simulink library "halout"  (R2021b)
settings: Solver=VariableStepAuto  StartTime=0.0  StopTime=10.0  RelTol=1e-3
undefined symbols (not defined in the file): C_TASK_5MS_S, FALSE, KHAL_CAN1FDAPS3E2E_flg, KHAL_CAN1FDAPS3TxReq_flg, KHAL_CAN1FDVCU2E2E_flg, KHAL_CAN1FDVCU2TxReq_flg, KHAL_CAN1FDVCU3E2E_flg, KHAL_CAN1FDVCU3TxReq_flg, KHAL_CAN1TxReq_flg, KHAL_CAN2TxReq_flg, KHAL_CAN3FDVCU1TxReq_flg, KHAL_CAN3FDVCU2E2E_flg, KHAL_CAN3FDVCU2TxReq_flg, KHAL_CAN3TxReq_flg, KHAL_CAN4FDVCU1E2E_flg, KHAL_CAN4FDVCU1TxReq_flg, KHAL_CAN4TxReq_flg, KHAL_CAN5TxReq_flg, ONE_INT, TRUE, ZERO_INT
libraries: FVT_lib x383, simulink x179
(part 1 of 20)
settings Model: Creator=13168  LastModifiedBy=yenst
settings SolverCC: AlgebraicLoopSolver=TrustRegion
settings DataIOCC: SaveFormat=Array  SignalLoggingSaveFormat=ModelDataLogs  ReturnWorkspaceOutputs=off
settings OptimizationCC: BlockReduction=off  BooleanDataType=off
settings DebuggingCC: SaveWithParameterizedLinksMsg=none  UnderspecifiedInitializationDetection=Classic  MergeDetectMultiDrivingBlocksExec=none  SignalResolutionControl=TryResolveAllWithWarning  SFMachineParentedDataDiag=warning
settings HardwareCC: TargetUnknown=on
settings ModelReferenceCC: PropagateSignalLabelsOutOfModel=off
settings ConfigComp: CovMetricSettings=dw  CovSaveCumulativeToWorkspaceVar=on  CovSaveSingleToWorkspaceVar=on

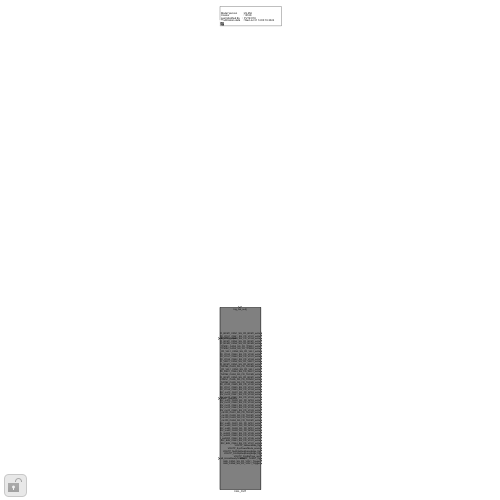
[thumbnail: Simulink's stored preview of the top-level diagram]
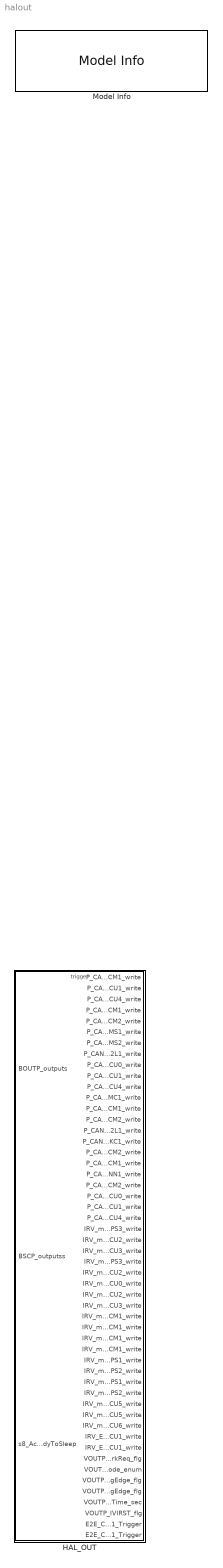
== system halout ==
  HAL_OUT : Subsystem
      settings: RTWSystemCode=Nonreusable function  RTWFcnNameOpts=Use subsystem name  RTWFileNameOpts=Use subsystem name
  Model Info : simulink/Model-Wide Utilities/Model Info  Frame=on  DisplayStringWithTags=|  HorizontalTextAlignment=Left  LeftAlignmentValue=0.02
      | Model Version        : %<ModelVersion>
      | Creator                   : %<Creator>
      | Last Modified By    : %<LastModifiedBy>
      | Modification date    : %<LastModificationDate>

== system halout/HAL_OUT ==
  BOUTP_outputs : Inport  OutDataTypeStr=Bus: BOUTP_outputs
  BSCP_outputss : Inport  Port=2  OutDataTypeStr=Bus:BSCP_outputs
  s8_AcoreReadyToSleep : Inport  Port=3
  trig_hal_out : TriggerPort  TriggerType=function-call  VariantControl=(inherit)
  Bus Selector : BusSelector  OutputSignals=VOUTP_AllCANTxReq_flg
  Bus_Selector : BusSelector  OutputSignals=VOUTP_NetworkReq_flg,VOUTP_SysPowerMode_enum,VOUTP_NvWriteReqRisingEdge_flg,VOUTP_FdcSlpReqRisingEdge_flg,VOUTP_FdcSlpTime_sec,VOUTP_IVIRST_flg
  CAN1 : Subsystem  TreatAsAtomicUnit=on
  CAN2 : Subsystem  TreatAsAtomicUnit=on
  CAN3 : Subsystem  TreatAsAtomicUnit=on
  CAN4 : Subsystem  TreatAsAtomicUnit=on
  CAN5 : Subsystem  TreatAsAtomicUnit=on
  CAN_Scheduler : Stateflow chart  TreatAsAtomicUnit=on
  Constant : Constant  Value=KHAL_CAN1TxReq_flg
  Constant1 : Constant  Value=KHAL_CAN2TxReq_flg
  Constant2 : Constant  Value=KHAL_CAN3TxReq_flg
  Constant3 : Constant  Value=KHAL_CAN4TxReq_flg
  Constant4 : Constant  Value=KHAL_CAN5TxReq_flg
  P_CAN1_FD_BCM1_CAN1_SG_FD_BCM1_write : Outport  OutDataTypeStr=Bus: DT_CAN1_SG_FD_BCM1
  P_CAN1_FD_VCU1_CAN1_SG_FD_VCU1_write : Outport  Port=2  OutDataTypeStr=Bus: DT_CAN1_SG_FD_VCU1
  P_CAN1_FD_VCU4_CAN1_SG_FD_VCU4_write : Outport  Port=3  OutDataTypeStr=Bus: DT_CAN1_SG_FD_VCU4
  P_CAN2_FD_BCM1_CAN2_SG_FD_BCM1_write : Outport  Port=4  OutDataTypeStr=Bus: DT_CAN2_SG_FD_BCM1
  P_CAN2_FD_BCM2_CAN2_SG_FD_BCM2_write : Outport  Port=5  OutDataTypeStr=Bus: DT_CAN2_SG_FD_BCM2
  P_CAN2_FD_TPMS1_CAN2_SG_FD_TPMS1_write : Outport  Port=6  OutDataTypeStr=Bus: DT_CAN2_SG_FD_TPMS1
  P_CAN2_FD_TPMS2_CAN2_SG_FD_TPMS2_write : Outport  Port=7  OutDataTypeStr=Bus: DT_CAN2_SG_FD_TPMS2
  P_CAN2_FD_V2L1_CAN2_SG_FD_V2L1_write : Outport  Port=8  OutDataTypeStr=Bus: DT_CAN2_SG_FD_V2L1
  P_CAN2_FD_VCU0_CAN2_SG_FD_VCU0_write : Outport  Port=9  OutDataTypeStr=Bus: DT_CAN2_SG_FD_VCU0
  P_CAN2_FD_VCU1_CAN2_SG_FD_VCU1_write : Outport  Port=10  OutDataTypeStr=Bus: DT_CAN2_SG_FD_VCU1
  P_CAN2_FD_VCU4_CAN2_SG_FD_VCU4_write : Outport  Port=11  OutDataTypeStr=Bus: DT_CAN2_SG_FD_VCU4
  P_CAN2_FD_VMC1_CAN2_SG_FD_VMC1_write : Outport  Port=12  OutDataTypeStr=Bus: DT_CAN2_SG_FD_VMC1
  P_CAN3_FD_BCM1_CAN3_SG_FD_BCM1_write : Outport  Port=13  OutDataTypeStr=Bus: DT_CAN3_SG_FD_BCM1
  P_CAN3_FD_THCM2_CAN3_SG_FD_THCM2_write : Outport  Port=14  OutDataTypeStr=Bus: DT_CAN3_SG_FD_THCM2
  P_CAN3_FD_V2L1_CAN3_SG_FD_V2L1_write : Outport  Port=15  OutDataTypeStr=Bus: DT_CAN3_SG_FD_V2L1
  P_CAN4_FD_DKC1_CAN4_SG_FD_DKC1_write : Outport  Port=16  OutDataTypeStr=Bus: DT_CAN4_SG_FD_DKC1
  P_CAN4_FD_THCM2_CAN4_SG_FD_THCM2_write : Outport  Port=17  OutDataTypeStr=Bus: DT_CAN4_SG_FD_THCM2
  P_CAN5_FD_BCM1_CAN5_SG_FD_BCM1_write : Outport  Port=18  OutDataTypeStr=Bus: DT_CAN5_SG_FD_BCM1
  P_CAN5_FD_CONN1_CAN5_SG_FD_CONN1_write : Outport  Port=19  OutDataTypeStr=Bus: DT_CAN5_SG_FD_CONN1
  P_CAN5_FD_THCM2_CAN5_SG_FD_THCM2_write : Outport  Port=20  OutDataTypeStr=Bus: DT_CAN5_SG_FD_THCM2
  P_CAN5_FD_VCU0_CAN5_SG_FD_VCU0_write : Outport  Port=21  OutDataTypeStr=Bus: DT_CAN5_SG_FD_VCU0
  P_CAN5_FD_VCU1_CAN5_SG_FD_VCU1_write : Outport  Port=22  OutDataTypeStr=Bus: DT_CAN5_SG_FD_VCU1
  P_CAN5_FD_VCU4_CAN5_SG_FD_VCU4_write : Outport  Port=23  OutDataTypeStr=Bus: DT_CAN5_SG_FD_VCU4
  IRV_ms10_CAN1_SG_FD_APS3_write : Outport  Port=24  OutDataTypeStr=Bus: DT_CAN1_SG_FD_APS3
  IRV_ms10_CAN1_SG_FD_VCU2_write : Outport  Port=25  OutDataTypeStr=Bus: DT_CAN1_SG_FD_VCU2
  IRV_ms10_CAN1_SG_FD_VCU3_write : Outport  Port=26  OutDataTypeStr=Bus: DT_CAN1_SG_FD_VCU3
  IRV_ms10_CAN2_SG_FD_APS3_write : Outport  Port=27  OutDataTypeStr=Bus: DT_CAN2_SG_FD_APS3
  IRV_ms10_CAN2_SG_FD_VCU2_write : Outport  Port=28  OutDataTypeStr=Bus: DT_CAN2_SG_FD_VCU2
  IRV_ms10_CAN3_SG_FD_VCU0_write : Outport  Port=29  OutDataTypeStr=Bus: DT_CAN3_SG_FD_VCU0
  IRV_ms10_CAN3_SG_FD_VCU2_write : Outport  Port=30  OutDataTypeStr=Bus: DT_CAN3_SG_FD_VCU2
  IRV_ms10_CAN5_SG_FD_VCU3_write : Outport  Port=31  OutDataTypeStr=Bus: DT_CAN5_SG_FD_VCU3
  IRV_ms100_CAN1_SG_FD_THCM1_write : Outport  Port=32  OutDataTypeStr=Bus: DT_CAN1_SG_FD_THCM1
  IRV_ms100_CAN2_SG_FD_THCM1_write : Outport  Port=33  OutDataTypeStr=Bus: DT_CAN2_SG_FD_THCM1
  IRV_ms100_CAN3_SG_FD_THCM1_write : Outport  Port=34  OutDataTypeStr=Bus: DT_CAN3_SG_FD_THCM1
  IRV_ms100_CAN4_SG_FD_THCM1_write : Outport  Port=35  OutDataTypeStr=Bus: DT_CAN4_SG_FD_THCM1
  IRV_ms20_CAN1_SG_FD_APS1_write : Outport  Port=36  OutDataTypeStr=Bus: DT_CAN1_SG_FD_APS1
  IRV_ms20_CAN1_SG_FD_APS2_write : Outport  Port=37  OutDataTypeStr=Bus: DT_CAN1_SG_FD_APS2
  IRV_ms20_CAN2_SG_FD_APS1_write : Outport  Port=38  OutDataTypeStr=Bus: DT_CAN2_SG_FD_APS1
  IRV_ms20_CAN2_SG_FD_APS2_write : Outport  Port=39  OutDataTypeStr=Bus: DT_CAN2_SG_FD_APS2
  IRV_ms500_CAN2_SG_FD_VCU5_write : Outport  Port=40  OutDataTypeStr=Bus: DT_CAN2_SG_FD_VCU5
  IRV_ms500_CAN5_SG_FD_VCU5_write : Outport  Port=41  OutDataTypeStr=Bus: DT_CAN5_SG_FD_VCU5
  IRV_ms5000_CAN2_SG_FD_VCU6_write : Outport  Port=42  OutDataTypeStr=Bus: DT_CAN2_SG_FD_VCU6
  IRV_E2E_CAN3_SG_FD_VCU1_write : Outport  Port=43  OutDataTypeStr=Bus: DT_CAN3_SG_FD_VCU1
  IRV_E2E_CAN4_SG_FD_VCU1_write : Outport  Port=44  OutDataTypeStr=Bus: DT_CAN4_SG_FD_VCU1
  VOUTP_NetworkReq_flg : Outport  Port=45
  VOUTP_SysPowerMode_enum : Outport  Port=46
  VOUTP_NvWriteReqRisingEdge_flg : Outport  Port=47
  VOUTP_FdcSlpReqRisingEdge_flg : Outport  Port=48
  VOUTP_FdcSlpTime_sec : Outport  Port=49
  VOUTP_IVIRST_flg : Outport  Port=50
  E2E_CAN3_SG_FD_VCU1_Trigger : Outport  Port=51
  E2E_CAN4_SG_FD_VCU1_Trigger : Outport  Port=52
  wires:
  BSCP_outputss/1 -> [BSCP_outputs]
  BOUTP_outputs/1 -> [BOUTP_outputs]
  Bus Selector/1 -> CAN_Scheduler/6(VOUTP_ALLCANTxReq_flg)  "<VOUTP_AllCANTxReq_flg>"
  [BOUTP_outputs] -> Bus Selector/1
  Constant1/1 -> CAN_Scheduler/2(KHAL_CAN2TxReq_flg)
  Constant3/1 -> CAN_Scheduler/4(KHAL_CAN4TxReq_flg)
  CAN_Scheduler/1(trig_can1()) -> [trig_can1]
  CAN_Scheduler/2(trig_can2()) -> [trig_can2]
  Constant/1 -> CAN_Scheduler/1(KHAL_CAN1TxReq_flg)
  CAN_Scheduler/4(trig_can4()) -> [trig_can4]
  CAN_Scheduler/5(trig_can5()) -> [trig_can5]
  Constant4/1 -> CAN_Scheduler/5(KHAL_CAN5TxReq_flg)
  Constant2/1 -> CAN_Scheduler/3(KHAL_CAN3TxReq_flg)
  CAN_Scheduler/3(trig_can3()) -> [trig_can3]
  [trig_can1] -> CAN1/Trigger
  [trig_can4] -> CAN4/Trigger
  [trig_can5] -> CAN5/Trigger
  [trig_can2] -> CAN2/Trigger
  [trig_can3] -> CAN3/Trigger
  CAN1/4(DT_CAN1_SG_FD_BCM1) -> P_CAN1_FD_BCM1_CAN1_SG_FD_BCM1_write/1
  CAN4/1(DT_CAN4_SG_FD_DKC1) -> P_CAN4_FD_DKC1_CAN4_SG_FD_DKC1_write/1
  Bus_Selector/4 -> VOUTP_FdcSlpReqRisingEdge_flg/1  "<VOUTP_FdcSlpReqRisingEdge_flg>"
  Bus_Selector/2 -> VOUTP_SysPowerMode_enum/1  "<VOUTP_SysPowerMode_enum>"
  Bus_Selector/1 -> VOUTP_NetworkReq_flg/1  "<VOUTP_NetworkReq_flg>"
  CAN3/7(DT_CAN3_SG_FD_VCU1) -> IRV_E2E_CAN3_SG_FD_VCU1_write/1
  CAN5/8(DT_CAN5_SG_FD_VCU5) -> IRV_ms500_CAN5_SG_FD_VCU5_write/1
  CAN1/1(DT_CAN1_SG_FD_APS1) -> IRV_ms20_CAN1_SG_FD_APS1_write/1
  CAN4/2(DT_CAN4_SG_FD_THCM1) -> IRV_ms100_CAN4_SG_FD_THCM1_write/1
  Bus_Selector/3 -> VOUTP_NvWriteReqRisingEdge_flg/1  "<VOUTP_NvWriteReqRisingEdge_flg>"
  CAN4/3(DT_CAN4_SG_FD_THCM2) -> P_CAN4_FD_THCM2_CAN4_SG_FD_THCM2_write/1
  CAN2/6(DT_CAN2_SG_FD_THCM1) -> IRV_ms100_CAN2_SG_FD_THCM1_write/1
  CAN3/4(DT_CAN3_SG_FD_V2L1) -> P_CAN3_FD_V2L1_CAN3_SG_FD_V2L1_write/1
  CAN3/8(DT_CAN3_SG_FD_VCU2) -> IRV_ms10_CAN3_SG_FD_VCU2_write/1
  s8_AcoreReadyToSleep/1 -> CAN3/3(s8_AcoreReadyToSleep)
  CAN3/5(DT_CAN3_SG_FD_VCU0) -> IRV_ms10_CAN3_SG_FD_VCU0_write/1
  CAN2/15(DT_CAN2_SG_FD_VCU6) -> IRV_ms5000_CAN2_SG_FD_VCU6_write/1
  CAN2/12(DT_CAN2_SG_FD_VCU2) -> IRV_ms10_CAN2_SG_FD_VCU2_write/1
  CAN1/2(DT_CAN1_SG_FD_APS2) -> IRV_ms20_CAN1_SG_FD_APS2_write/1
  CAN2/3(DT_CAN2_SG_FD_APS3) -> IRV_ms10_CAN2_SG_FD_APS3_write/1
  CAN1/8(DT_CAN1_SG_FD_VCU3) -> IRV_ms10_CAN1_SG_FD_VCU3_write/1
  CAN5/5(DT_CAN5_SG_FD_VCU1) -> P_CAN5_FD_VCU1_CAN5_SG_FD_VCU1_write/1
  CAN2/9(DT_CAN2_SG_FD_V2L1) -> P_CAN2_FD_V2L1_CAN2_SG_FD_V2L1_write/1
  CAN1/5(DT_CAN1_SG_FD_THCM1) -> IRV_ms100_CAN1_SG_FD_THCM1_write/1
  CAN2/5(DT_CAN2_SG_FD_BCM2) -> P_CAN2_FD_BCM2_CAN2_SG_FD_BCM2_write/1
  CAN2/4(DT_CAN2_SG_FD_BCM1) -> P_CAN2_FD_BCM1_CAN2_SG_FD_BCM1_write/1
  CAN1/9(DT_CAN1_SG_FD_VCU4) -> P_CAN1_FD_VCU4_CAN1_SG_FD_VCU4_write/1
  CAN2/2(DT_CAN2_SG_FD_APS2) -> IRV_ms20_CAN2_SG_FD_APS2_write/1
  CAN3/3(DT_CAN3_SG_FD_THCM2) -> P_CAN3_FD_THCM2_CAN3_SG_FD_THCM2_write/1
  CAN2/14(DT_CAN2_SG_FD_VCU5) -> IRV_ms500_CAN2_SG_FD_VCU5_write/1
  CAN3/1(DT_CAN3_SG_FD_BCM1) -> P_CAN3_FD_BCM1_CAN3_SG_FD_BCM1_write/1
  CAN2/13(DT_CAN2_SG_FD_VCU4) -> P_CAN2_FD_VCU4_CAN2_SG_FD_VCU4_write/1
  CAN2/11(DT_CAN2_SG_FD_VCU1) -> P_CAN2_FD_VCU1_CAN2_SG_FD_VCU1_write/1
  CAN2/10(DT_CAN2_SG_FD_VCU0) -> P_CAN2_FD_VCU0_CAN2_SG_FD_VCU0_write/1
  CAN1/6(DT_CAN1_SG_FD_VCU1) -> P_CAN1_FD_VCU1_CAN1_SG_FD_VCU1_write/1
  Bus_Selector/5 -> VOUTP_FdcSlpTime_sec/1  "<VOUTP_FdcSlpTime_sec>"
  CAN2/7(DT_CAN2_SG_FD_TPMS1) -> P_CAN2_FD_TPMS1_CAN2_SG_FD_TPMS1_write/1
  CAN2/1(DT_CAN2_SG_FD_APS1) -> IRV_ms20_CAN2_SG_FD_APS1_write/1
  [BSCP_outputs] -> CAN5/2(BSCP_outputs)
  CAN5/4(DT_CAN5_SG_FD_VCU0) -> P_CAN5_FD_VCU0_CAN5_SG_FD_VCU0_write/1
  [BSCP_outputs] -> CAN4/2(BSCP_outputs)
  [BOUTP_outputs] -> CAN5/1(BOUTP_outputs)
  CAN2/16(DT_CAN2_SG_FD_VMC1) -> P_CAN2_FD_VMC1_CAN2_SG_FD_VMC1_write/1
  CAN5/2(DT_CAN5_SG_FD_CONN1) -> P_CAN5_FD_CONN1_CAN5_SG_FD_CONN1_write/1
  [BOUTP_outputs] -> CAN4/1(BOUTP_outputs)
  CAN2/8(DT_CAN2_SG_FD_TPMS2) -> P_CAN2_FD_TPMS2_CAN2_SG_FD_TPMS2_write/1
  CAN4/4(E2E_CAN4_SG_FD_VCU1_Trigger) -> E2E_CAN4_SG_FD_VCU1_Trigger/1
  CAN5/6(DT_CAN5_SG_FD_VCU3) -> IRV_ms10_CAN5_SG_FD_VCU3_write/1
  CAN5/3(DT_CAN5_SG_FD_THCM2) -> P_CAN5_FD_THCM2_CAN5_SG_FD_THCM2_write/1
  [BOUTP_outputs] -> CAN3/1(BOUTP_outputs)
  CAN3/6(E2E_CAN3_SG_FD_VCU1_Trigger) -> E2E_CAN3_SG_FD_VCU1_Trigger/1
  [BSCP_outputs] -> CAN3/2(BSCP_outputs)
  CAN3/2(DT_CAN3_SG_FD_THCM1) -> IRV_ms100_CAN3_SG_FD_THCM1_write/1
  [BSCP_outputs] -> CAN2/2(BSCP_outputs)
  [BSCP_outputs] -> CAN1/2(BSCP_outputs)
  CAN5/7(DT_CAN5_SG_FD_VCU4) -> P_CAN5_FD_VCU4_CAN5_SG_FD_VCU4_write/1
  CAN5/1(DT_CAN5_SG_FD_BCM1) -> P_CAN5_FD_BCM1_CAN5_SG_FD_BCM1_write/1
  [BOUTP_outputs] -> CAN1/1(BOUTP_outputs)
  CAN4/5(DT_CAN4_SG_FD_VCU1) -> IRV_E2E_CAN4_SG_FD_VCU1_write/1
  [BOUTP_outputs] -> Bus_Selector/1
  [BOUTP_outputs] -> CAN2/1(BOUTP_outputs)
  CAN1/3(DT_CAN1_SG_FD_APS3) -> IRV_ms10_CAN1_SG_FD_APS3_write/1
  Bus_Selector/6 -> VOUTP_IVIRST_flg/1  "<VOUTP_IVIRST_flg>"
  CAN1/7(DT_CAN1_SG_FD_VCU2) -> IRV_ms10_CAN1_SG_FD_VCU2_write/1

== system halout/HAL_OUT/CAN1 ==
  BOUTP_outputs : Inport  OutDataTypeStr=Bus: BOUTP_outputs
  BSCP_outputs : Inport  Port=2  OutDataTypeStr=Bus: BSCP_outputs
  Trigger : TriggerPort  TriggerType=function-call  VariantControl=(inherit)
  Constant : Constant  Value=KHAL_CAN1FDAPS3TxReq_flg
  Constant1 : Constant  Value=KHAL_CAN1FDVCU2TxReq_flg
  Constant2 : Constant  Value=KHAL_CAN1FDVCU3TxReq_flg
  FD_APS1_0x236 : Subsystem
  FD_APS2_0x210 : Subsystem
  FD_APS3_0x238 : Subsystem  TreatAsAtomicUnit=on
  FD_APS3_Tx : Subsystem  AncestorBlock=FVT_lib/hal/MsgTxController  mask{CycleTime=10}
      mask prompts: CycleTime "MsgCycleTime_ms"
      mask help: MeasumentTrigerTime
      mask Display: fprintf('Tx Method: Cycle\nMsg Cycletime ms: %3.0f', CycleTime);
  FD_BCM1_0x216 : Subsystem
  FD_THCM1_0x182 : Subsystem
  FD_VCU1_0x116 : Subsystem
  FD_VCU2_0x154 : Subsystem  TreatAsAtomicUnit=on
  FD_VCU2_Tx : Subsystem  AncestorBlock=FVT_lib/hal/MsgTxController  mask{CycleTime=10}
      mask prompts: CycleTime "MsgCycleTime_ms"
      mask help: MeasumentTrigerTime
      mask Display: fprintf('Tx Method: Cycle\nMsg Cycletime ms: %3.0f', CycleTime);
  FD_VCU3_0x159 : Subsystem  TreatAsAtomicUnit=on
  FD_VCU3_Tx : Subsystem  AncestorBlock=FVT_lib/hal/MsgTxController  mask{CycleTime=10}
      mask prompts: CycleTime "MsgCycleTime_ms"
      mask help: MeasumentTrigerTime
      mask Display: fprintf('Tx Method: Cycle\nMsg Cycletime ms: %3.0f', CycleTime);
  FD_VCU4_0x3C0 : Subsystem
  DT_CAN1_SG_FD_APS1 : Outport  OutDataTypeStr=Bus: DT_CAN1_SG_FD_APS1
  DT_CAN1_SG_FD_APS2 : Outport  Port=2  OutDataTypeStr=Bus: DT_CAN1_SG_FD_APS2
  DT_CAN1_SG_FD_APS3 : Outport  Port=3  OutDataTypeStr=Bus: DT_CAN1_SG_FD_APS3
  DT_CAN1_SG_FD_BCM1 : Outport  Port=4  OutDataTypeStr=Bus: DT_CAN1_SG_FD_BCM1
  DT_CAN1_SG_FD_THCM1 : Outport  Port=5  OutDataTypeStr=Bus: DT_CAN1_SG_FD_THCM1
  DT_CAN1_SG_FD_VCU1 : Outport  Port=6  OutDataTypeStr=Bus: DT_CAN1_SG_FD_VCU1
  DT_CAN1_SG_FD_VCU2 : Outport  Port=7  OutDataTypeStr=Bus: DT_CAN1_SG_FD_VCU2
  DT_CAN1_SG_FD_VCU3 : Outport  Port=8  OutDataTypeStr=Bus: DT_CAN1_SG_FD_VCU3
  DT_CAN1_SG_FD_VCU4 : Outport  Port=9  OutDataTypeStr=Bus: DT_CAN1_SG_FD_VCU4
  wires:
  BOUTP_outputs/1 -> [BOUTP_outputs]
  BSCP_outputs/1 -> [BSCP_outputs]
  [BSCP_outputs] -> FD_APS1_0x236/1(BSCP_outputs)
  [BOUTP_outputs] -> FD_APS1_0x236/2(BOUTP_outputs)
  FD_APS1_0x236/1(FD_APS1) -> DT_CAN1_SG_FD_APS1/1
  [BSCP_outputs] -> FD_APS2_0x210/1(BSCP_outputs)
  [BOUTP_outputs] -> FD_APS2_0x210/2(BOUTP_outputs)
  FD_APS2_0x210/1(FD_APS2) -> DT_CAN1_SG_FD_APS2/1
  [BSCP_outputs] -> FD_APS3_0x238/1(BSCP_outputs)
  [BOUTP_outputs] -> FD_APS3_0x238/2(BOUTP_outputs)
  FD_APS3_Tx/1(TxTrigger) -> FD_APS3_0x238/Trigger
  Constant/1 -> FD_APS3_Tx/1(TxReq)
  FD_APS3_0x238/1(FD_APS3) -> DT_CAN1_SG_FD_APS3/1
  [BSCP_outputs] -> FD_BCM1_0x216/1(BSCP_outputs)
  [BOUTP_outputs] -> FD_BCM1_0x216/2(BOUTP_outputs)
  FD_BCM1_0x216/1(FD_BCM1) -> DT_CAN1_SG_FD_BCM1/1
  [BSCP_outputs] -> FD_THCM1_0x182/1(BSCP_outputs)
  [BOUTP_outputs] -> FD_THCM1_0x182/2(BOUTP_outputs)
  FD_THCM1_0x182/1(FD_THCM1) -> DT_CAN1_SG_FD_THCM1/1
  [BSCP_outputs] -> FD_VCU1_0x116/1(BSCP_outputs)
  [BOUTP_outputs] -> FD_VCU1_0x116/2(BOUTP_outputs)
  FD_VCU1_0x116/1(FD_VCU1) -> DT_CAN1_SG_FD_VCU1/1
  [BSCP_outputs] -> FD_VCU2_0x154/1(BSCP_outputs)
  [BOUTP_outputs] -> FD_VCU2_0x154/2(BOUTP_outputs)
  FD_VCU2_Tx/1(TxTrigger) -> FD_VCU2_0x154/Trigger
  Constant1/1 -> FD_VCU2_Tx/1(TxReq)
  FD_VCU2_0x154/1(FD_VCU2) -> DT_CAN1_SG_FD_VCU2/1
  [BSCP_outputs] -> FD_VCU3_0x159/1(BSCP_outputs)
  [BOUTP_outputs] -> FD_VCU3_0x159/2(BOUTP_outputs)
  FD_VCU3_Tx/1(TxTrigger) -> FD_VCU3_0x159/Trigger
  Constant2/1 -> FD_VCU3_Tx/1(TxReq)
  FD_VCU3_0x159/1(FD_VCU3) -> DT_CAN1_SG_FD_VCU3/1
  [BSCP_outputs] -> FD_VCU4_0x3C0/1(BSCP_outputs)
  [BOUTP_outputs] -> FD_VCU4_0x3C0/2(BOUTP_outputs)
  FD_VCU4_0x3C0/1(FD_VCU4) -> DT_CAN1_SG_FD_VCU4/1

== system halout/HAL_OUT/CAN2 ==
  BOUTP_outputs : Inport  OutDataTypeStr=Bus: BOUTP_outputs
  BSCP_outputs : Inport  Port=2  OutDataTypeStr=Bus: BSCP_outputs
  Trigger : TriggerPort  TriggerType=function-call  VariantControl=(inherit)
  FD_APS1_0x236 : Subsystem
  FD_APS2_0x210 : Subsystem
  FD_APS3_0x238 : Subsystem
  FD_BCM1_0x216 : Subsystem
  FD_BCM2_0x217 : Subsystem
  FD_THCM1_0x182 : Subsystem
  FD_TPMS1_0x435 : Subsystem
  FD_TPMS2_0x436 : Subsystem
  FD_V2L1_0x374 : Subsystem
  FD_VCU0_0x1F0 : Subsystem
  FD_VCU1_0x116 : Subsystem
  FD_VCU2_0x154 : Subsystem
  FD_VCU4_0x3C0 : Subsystem
  FD_VCU5_0x245 : Subsystem
  FD_VCU6_0x3C3 : Subsystem
  FD_VMC1_0x17F : Subsystem
  DT_CAN2_SG_FD_APS1 : Outport  OutDataTypeStr=Bus: DT_CAN2_SG_FD_APS1
  DT_CAN2_SG_FD_APS2 : Outport  Port=2  OutDataTypeStr=Bus: DT_CAN2_SG_FD_APS2
  DT_CAN2_SG_FD_APS3 : Outport  Port=3  OutDataTypeStr=Bus: DT_CAN2_SG_FD_APS3
  DT_CAN2_SG_FD_BCM1 : Outport  Port=4  OutDataTypeStr=Bus: DT_CAN2_SG_FD_BCM1
  DT_CAN2_SG_FD_BCM2 : Outport  Port=5  OutDataTypeStr=Bus: DT_CAN2_SG_FD_BCM2
  DT_CAN2_SG_FD_THCM1 : Outport  Port=6  OutDataTypeStr=Bus: DT_CAN2_SG_FD_THCM1
  DT_CAN2_SG_FD_TPMS1 : Outport  Port=7  OutDataTypeStr=Bus: DT_CAN2_SG_FD_TPMS1
  DT_CAN2_SG_FD_TPMS2 : Outport  Port=8  OutDataTypeStr=Bus: DT_CAN2_SG_FD_TPMS2
  DT_CAN2_SG_FD_V2L1 : Outport  Port=9  OutDataTypeStr=Bus: DT_CAN2_SG_FD_V2L1
  DT_CAN2_SG_FD_VCU0 : Outport  Port=10  OutDataTypeStr=Bus: DT_CAN2_SG_FD_VCU0
  DT_CAN2_SG_FD_VCU1 : Outport  Port=11  OutDataTypeStr=Bus: DT_CAN2_SG_FD_VCU1
  DT_CAN2_SG_FD_VCU2 : Outport  Port=12  OutDataTypeStr=Bus: DT_CAN2_SG_FD_VCU2
  DT_CAN2_SG_FD_VCU4 : Outport  Port=13  OutDataTypeStr=Bus: DT_CAN2_SG_FD_VCU4
  DT_CAN2_SG_FD_VCU5 : Outport  Port=14  OutDataTypeStr=Bus: DT_CAN2_SG_FD_VCU5
  DT_CAN2_SG_FD_VCU6 : Outport  Port=15  OutDataTypeStr=Bus: DT_CAN2_SG_FD_VCU6
  DT_CAN2_SG_FD_VMC1 : Outport  Port=16  OutDataTypeStr=Bus: DT_CAN2_SG_FD_VMC1
  wires:
  BOUTP_outputs/1 -> [BOUTP_outputs]
  BSCP_outputs/1 -> [BSCP_outputs]
  [BSCP_outputs] -> FD_APS1_0x236/1(BSCP_outputs)
  [BOUTP_outputs] -> FD_APS1_0x236/2(BOUTP_outputs)
  FD_APS1_0x236/1(FD_APS1) -> DT_CAN2_SG_FD_APS1/1
  [BSCP_outputs] -> FD_APS2_0x210/1(BSCP_outputs)
  [BOUTP_outputs] -> FD_APS2_0x210/2(BOUTP_outputs)
  FD_APS2_0x210/1(FD_APS2) -> DT_CAN2_SG_FD_APS2/1
  [BSCP_outputs] -> FD_APS3_0x238/1(BSCP_outputs)
  [BOUTP_outputs] -> FD_APS3_0x238/2(BOUTP_outputs)
  FD_APS3_0x238/1(FD_APS3) -> DT_CAN2_SG_FD_APS3/1
  [BSCP_outputs] -> FD_BCM1_0x216/1(BSCP_outputs)
  [BOUTP_outputs] -> FD_BCM1_0x216/2(BOUTP_outputs)
  FD_BCM1_0x216/1(FD_BCM1) -> DT_CAN2_SG_FD_BCM1/1
  [BSCP_outputs] -> FD_BCM2_0x217/1(BSCP_outputs)
  [BOUTP_outputs] -> FD_BCM2_0x217/2(BOUTP_outputs)
  FD_BCM2_0x217/1(FD_BCM2) -> DT_CAN2_SG_FD_BCM2/1
  [BSCP_outputs] -> FD_THCM1_0x182/1(BSCP_outputs)
  [BOUTP_outputs] -> FD_THCM1_0x182/2(BOUTP_outputs)
  FD_THCM1_0x182/1(FD_THCM1) -> DT_CAN2_SG_FD_THCM1/1
  [BSCP_outputs] -> FD_TPMS1_0x435/1(BSCP_outputs)
  [BOUTP_outputs] -> FD_TPMS1_0x435/2(BOUTP_outputs)
  FD_TPMS1_0x435/1(FD_TPMS1) -> DT_CAN2_SG_FD_TPMS1/1
  [BSCP_outputs] -> FD_TPMS2_0x436/1(BSCP_outputs)
  [BOUTP_outputs] -> FD_TPMS2_0x436/2(BOUTP_outputs)
  FD_TPMS2_0x436/1(FD_TPMS2) -> DT_CAN2_SG_FD_TPMS2/1
  [BSCP_outputs] -> FD_V2L1_0x374/1(BSCP_outputs)
  [BOUTP_outputs] -> FD_V2L1_0x374/2(BOUTP_outputs)
  FD_V2L1_0x374/1(FD_V2L1) -> DT_CAN2_SG_FD_V2L1/1
  [BSCP_outputs] -> FD_VCU0_0x1F0/1(BSCP_outputs)
  [BOUTP_outputs] -> FD_VCU0_0x1F0/2(BOUTP_outputs)
  FD_VCU0_0x1F0/1(FD_VCU0) -> DT_CAN2_SG_FD_VCU0/1
  [BSCP_outputs] -> FD_VCU1_0x116/1(BSCP_outputs)
  [BOUTP_outputs] -> FD_VCU1_0x116/2(BOUTP_outputs)
  FD_VCU1_0x116/1(FD_VCU1) -> DT_CAN2_SG_FD_VCU1/1
  [BSCP_outputs] -> FD_VCU2_0x154/1(BSCP_outputs)
  [BOUTP_outputs] -> FD_VCU2_0x154/2(BOUTP_outputs)
  FD_VCU2_0x154/1(FD_VCU2) -> DT_CAN2_SG_FD_VCU2/1
  [BSCP_outputs] -> FD_VCU4_0x3C0/1(BSCP_outputs)
  [BOUTP_outputs] -> FD_VCU4_0x3C0/2(BOUTP_outputs)
  FD_VCU4_0x3C0/1(FD_VCU4) -> DT_CAN2_SG_FD_VCU4/1
  [BSCP_outputs] -> FD_VCU5_0x245/1(BSCP_outputs)
  [BOUTP_outputs] -> FD_VCU5_0x245/2(BOUTP_outputs)
  FD_VCU5_0x245/1(FD_VCU5) -> DT_CAN2_SG_FD_VCU5/1
  [BSCP_outputs] -> FD_VCU6_0x3C3/1(BSCP_outputs)
  [BOUTP_outputs] -> FD_VCU6_0x3C3/2(BOUTP_outputs)
  FD_VCU6_0x3C3/1(FD_VCU6) -> DT_CAN2_SG_FD_VCU6/1
  [BSCP_outputs] -> FD_VMC1_0x17F/1(BSCP_outputs)
  [BOUTP_outputs] -> FD_VMC1_0x17F/2(BOUTP_outputs)
  FD_VMC1_0x17F/1(FD_VMC1) -> DT_CAN2_SG_FD_VMC1/1

== system halout/HAL_OUT/CAN3 ==
  BOUTP_outputs : Inport  OutDataTypeStr=Bus: BOUTP_outputs
  BSCP_outputs : Inport  Port=2  OutDataTypeStr=Bus: BSCP_outputs
  s8_AcoreReadyToSleep : Inport  Port=3
  Trigger : TriggerPort  TriggerType=function-call  VariantControl=(inherit)
  Constant : Constant  Value=KHAL_CAN3FDVCU1TxReq_flg
  Constant1 : Constant  Value=KHAL_CAN3FDVCU2TxReq_flg
  FD_BCM1_0x216 : Subsystem
  FD_THCM1_0x182 : Subsystem
  FD_THCM2_0x186 : Subsystem
  FD_V2L1_0x374 : Subsystem
  FD_VCU0_0x1F0 : Subsystem
  FD_VCU1_0x116 : Subsystem
  FD_VCU1_Tx : Subsystem  AncestorBlock=FVT_lib/hal/MsgTxController_CE  mask{CycleTime=100}
      mask prompts: CycleTime "MsgCycleTime_ms"
      mask help: MeasumentTrigerTime
      mask Display: fprintf('Tx Method: CE\nMsg Cycletime ms: %3.0f', CycleTime);
  FD_VCU2_0x154 : Subsystem  TreatAsAtomicUnit=on
  FD_VCU2_Tx : Subsystem  AncestorBlock=FVT_lib/hal/MsgTxController  mask{CycleTime=10}
      mask prompts: CycleTime "MsgCycleTime_ms"
      mask help: MeasumentTrigerTime
      mask Display: fprintf('Tx Method: Cycle\nMsg Cycletime ms: %3.0f', CycleTime);
  DT_CAN3_SG_FD_BCM1 : Outport  OutDataTypeStr=Bus: DT_CAN3_SG_FD_BCM1
  DT_CAN3_SG_FD_THCM1 : Outport  Port=2  OutDataTypeStr=Bus: DT_CAN3_SG_FD_THCM1
  DT_CAN3_SG_FD_THCM2 : Outport  Port=3  OutDataTypeStr=Bus: DT_CAN3_SG_FD_THCM2
  DT_CAN3_SG_FD_V2L1 : Outport  Port=4  OutDataTypeStr=Bus: DT_CAN3_SG_FD_V2L1
  DT_CAN3_SG_FD_VCU0 : Outport  Port=5  OutDataTypeStr=Bus: DT_CAN3_SG_FD_VCU0
  E2E_CAN3_SG_FD_VCU1_Trigger : Outport  Port=6
  DT_CAN3_SG_FD_VCU1 : Outport  Port=7  OutDataTypeStr=Bus: DT_CAN3_SG_FD_VCU1
  DT_CAN3_SG_FD_VCU2 : Outport  Port=8  OutDataTypeStr=Bus: DT_CAN3_SG_FD_VCU2
  wires:
  BOUTP_outputs/1 -> [BOUTP_outputs]
  BSCP_outputs/1 -> [BSCP_outputs]
  [BSCP_outputs] -> FD_BCM1_0x216/1(BSCP_outputs)
  [BOUTP_outputs] -> FD_BCM1_0x216/2(BOUTP_outputs)
  FD_BCM1_0x216/1(FD_BCM1) -> DT_CAN3_SG_FD_BCM1/1
  [BSCP_outputs] -> FD_THCM1_0x182/1(BSCP_outputs)
  [BOUTP_outputs] -> FD_THCM1_0x182/2(BOUTP_outputs)
  FD_THCM1_0x182/1(FD_THCM1) -> DT_CAN3_SG_FD_THCM1/1
  [BSCP_outputs] -> FD_THCM2_0x186/1(BSCP_outputs)
  [BOUTP_outputs] -> FD_THCM2_0x186/2(BOUTP_outputs)
  FD_THCM2_0x186/1(FD_THCM2) -> DT_CAN3_SG_FD_THCM2/1
  [BSCP_outputs] -> FD_V2L1_0x374/1(BSCP_outputs)
  [BOUTP_outputs] -> FD_V2L1_0x374/2(BOUTP_outputs)
  FD_V2L1_0x374/1(FD_V2L1) -> DT_CAN3_SG_FD_V2L1/1
  [BSCP_outputs] -> FD_VCU0_0x1F0/1(BSCP_outputs)
  [BOUTP_outputs] -> FD_VCU0_0x1F0/2(BOUTP_outputs)
  FD_VCU0_0x1F0/1(FD_VCU0) -> DT_CAN3_SG_FD_VCU0/1
  [BSCP_outputs] -> FD_VCU1_0x116/1(BSCP_outputs)
  [BOUTP_outputs] -> FD_VCU1_0x116/2(BOUTP_outputs)
  FD_VCU1_Tx/1(TxTrigger) -> E2E_CAN3_SG_FD_VCU1_Trigger/1
  Constant/1 -> FD_VCU1_Tx/1(TxReq)
  [BSCP_outputs] -> FD_VCU1_Tx/2(BSCP_outputs)
  [BOUTP_outputs] -> FD_VCU1_Tx/3(BOUTP_outputs)
  FD_VCU1_0x116/1(FD_VCU1) -> DT_CAN3_SG_FD_VCU1/1
  [BSCP_outputs] -> FD_VCU2_0x154/1(BSCP_outputs)
  [BOUTP_outputs] -> FD_VCU2_0x154/2(BOUTP_outputs)
  FD_VCU2_Tx/1(TxTrigger) -> FD_VCU2_0x154/Trigger
  Constant1/1 -> FD_VCU2_Tx/1(TxReq)
  FD_VCU2_0x154/1(FD_VCU2) -> DT_CAN3_SG_FD_VCU2/1
  s8_AcoreReadyToSleep/1 -> FD_VCU0_0x1F0/3(s8_AcoreReadyToSleep)

== system halout/HAL_OUT/CAN4 ==
  BOUTP_outputs : Inport  OutDataTypeStr=Bus: BOUTP_outputs
  BSCP_outputs : Inport  Port=2  OutDataTypeStr=Bus: BSCP_outputs
  Trigger : TriggerPort  TriggerType=function-call  VariantControl=(inherit)
  Constant : Constant  Value=KHAL_CAN4FDVCU1TxReq_flg
  Detect Change : simulink/Logic and Bit Operations/Detect Change  vinit=0  OutDataTypeStr=boolean
  FD_DKC1_0x253 : Subsystem
  FD_THCM1_0x182 : Subsystem
  FD_THCM2_0x186 : Subsystem
  FD_VCU1_0x116 : Subsystem  TreatAsAtomicUnit=on
  FD_VCU1_Tx : Subsystem  AncestorBlock=FVT_lib/hal/MsgTxController_CE  mask{CycleTime=100}
      mask prompts: CycleTime "MsgCycleTime_ms"
      mask help: MeasumentTrigerTime
      mask Display: fprintf('Tx Method: CE\nMsg Cycletime ms: %3.0f', CycleTime);
  Function-Call Subsystem : Subsystem  TreatAsAtomicUnit=on
  Unit Delay : UnitDelay  SampleTime=-1  HasFrameUpgradeWarning=on
  DT_CAN4_SG_FD_DKC1 : Outport  OutDataTypeStr=Bus: DT_CAN4_SG_FD_DKC1
  DT_CAN4_SG_FD_THCM1 : Outport  Port=2  OutDataTypeStr=Bus: DT_CAN4_SG_FD_THCM1
  DT_CAN4_SG_FD_THCM2 : Outport  Port=3  OutDataTypeStr=Bus: DT_CAN4_SG_FD_THCM2
  E2E_CAN4_SG_FD_VCU1_Trigger : Outport  Port=4
  DT_CAN4_SG_FD_VCU1 : Outport  Port=5  OutDataTypeStr=Bus: DT_CAN4_SG_FD_VCU1
  wires:
  BOUTP_outputs/1 -> [BOUTP_outputs]
  BSCP_outputs/1 -> [BSCP_outputs]
  [BSCP_outputs] -> FD_DKC1_0x253/1(BSCP_outputs)
  [BOUTP_outputs] -> FD_DKC1_0x253/2(BOUTP_outputs)
  FD_DKC1_0x253/1(FD_DKC1) -> DT_CAN4_SG_FD_DKC1/1
  [BSCP_outputs] -> FD_THCM1_0x182/1(BSCP_outputs)
  [BOUTP_outputs] -> FD_THCM1_0x182/2(BOUTP_outputs)
  FD_THCM1_0x182/1(FD_THCM1) -> DT_CAN4_SG_FD_THCM1/1
  [BSCP_outputs] -> FD_THCM2_0x186/1(BSCP_outputs)
  [BOUTP_outputs] -> FD_THCM2_0x186/2(BOUTP_outputs)
  FD_THCM2_0x186/1(FD_THCM2) -> DT_CAN4_SG_FD_THCM2/1
  [BSCP_outputs] -> FD_VCU1_0x116/1(BSCP_outputs)
  [BOUTP_outputs] -> FD_VCU1_0x116/2(BOUTP_outputs)
  Constant/1 -> FD_VCU1_Tx/1(TxReq)
  [BSCP_outputs] -> FD_VCU1_Tx/2(BSCP_outputs)
  [BOUTP_outputs] -> FD_VCU1_Tx/3(BOUTP_outputs)
  FD_VCU1_0x116/1(FD_VCU1) -> DT_CAN4_SG_FD_VCU1/1
  Unit Delay/1 -> E2E_CAN4_SG_FD_VCU1_Trigger/1
  Detect Change/1 -> Unit Delay/1
  Function-Call Subsystem/1(TriggerCAN4VCU1_CNT) -> Detect Change/1
  FD_VCU1_Tx/1(TriggerDataUpdate) -> FD_VCU1_0x116/Trigger
  FD_VCU1_Tx/2(TriggerCallCDD) -> Function-Call Subsystem/Trigger

== system halout/HAL_OUT/CAN5 ==
  BOUTP_outputs : Inport  OutDataTypeStr=Bus: BOUTP_outputs
  BSCP_outputs : Inport  Port=2  OutDataTypeStr=Bus: BSCP_outputs
  Trigger : TriggerPort  TriggerType=function-call  VariantControl=(inherit)
  FD_BCM1_0x216 : Subsystem
  FD_CONN1_0x43C : Subsystem
  FD_THCM2_0x186 : Subsystem
  FD_VCU0_0x1F0 : Subsystem
  FD_VCU1_0x116 : Subsystem
  FD_VCU3_0x159 : Subsystem
  FD_VCU4_0x3C0 : Subsystem
  FD_VCU5_0x245 : Subsystem
  DT_CAN5_SG_FD_BCM1 : Outport  OutDataTypeStr=Bus: DT_CAN5_SG_FD_BCM1
  DT_CAN5_SG_FD_CONN1 : Outport  Port=2  OutDataTypeStr=Bus: DT_CAN5_SG_FD_CONN1
  DT_CAN5_SG_FD_THCM2 : Outport  Port=3  OutDataTypeStr=Bus: DT_CAN5_SG_FD_THCM2
  DT_CAN5_SG_FD_VCU0 : Outport  Port=4  OutDataTypeStr=Bus: DT_CAN5_SG_FD_VCU0
  DT_CAN5_SG_FD_VCU1 : Outport  Port=5  OutDataTypeStr=Bus: DT_CAN5_SG_FD_VCU1
  DT_CAN5_SG_FD_VCU3 : Outport  Port=6  OutDataTypeStr=Bus: DT_CAN5_SG_FD_VCU3
  DT_CAN5_SG_FD_VCU4 : Outport  Port=7  OutDataTypeStr=Bus: DT_CAN5_SG_FD_VCU4
  DT_CAN5_SG_FD_VCU5 : Outport  Port=8  OutDataTypeStr=Bus: DT_CAN5_SG_FD_VCU5
  wires:
  BOUTP_outputs/1 -> [BOUTP_outputs]
  BSCP_outputs/1 -> [BSCP_outputs]
  [BSCP_outputs] -> FD_BCM1_0x216/1(BSCP_outputs)
  [BOUTP_outputs] -> FD_BCM1_0x216/2(BOUTP_outputs)
  FD_BCM1_0x216/1(FD_BCM1) -> DT_CAN5_SG_FD_BCM1/1
  [BSCP_outputs] -> FD_CONN1_0x43C/1(BSCP_outputs)
  [BOUTP_outputs] -> FD_CONN1_0x43C/2(BOUTP_outputs)
  FD_CONN1_0x43C/1(FD_CONN1) -> DT_CAN5_SG_FD_CONN1/1
  [BSCP_outputs] -> FD_THCM2_0x186/1(BSCP_outputs)
  [BOUTP_outputs] -> FD_THCM2_0x186/2(BOUTP_outputs)
  FD_THCM2_0x186/1(FD_THCM2) -> DT_CAN5_SG_FD_THCM2/1
  [BSCP_outputs] -> FD_VCU0_0x1F0/1(BSCP_outputs)
  [BOUTP_outputs] -> FD_VCU0_0x1F0/2(BOUTP_outputs)
  FD_VCU0_0x1F0/1(FD_VCU0) -> DT_CAN5_SG_FD_VCU0/1
  [BSCP_outputs] -> FD_VCU1_0x116/1(BSCP_outputs)
  [BOUTP_outputs] -> FD_VCU1_0x116/2(BOUTP_outputs)
  FD_VCU1_0x116/1(FD_VCU1) -> DT_CAN5_SG_FD_VCU1/1
  [BSCP_outputs] -> FD_VCU3_0x159/1(BSCP_outputs)
  [BOUTP_outputs] -> FD_VCU3_0x159/2(BOUTP_outputs)
  FD_VCU3_0x159/1(FD_VCU3) -> DT_CAN5_SG_FD_VCU3/1
  [BSCP_outputs] -> FD_VCU4_0x3C0/1(BSCP_outputs)
  [BOUTP_outputs] -> FD_VCU4_0x3C0/2(BOUTP_outputs)
  FD_VCU4_0x3C0/1(FD_VCU4) -> DT_CAN5_SG_FD_VCU4/1
  [BSCP_outputs] -> FD_VCU5_0x245/1(BSCP_outputs)
  [BOUTP_outputs] -> FD_VCU5_0x245/2(BOUTP_outputs)
  FD_VCU5_0x245/1(FD_VCU5) -> DT_CAN5_SG_FD_VCU5/1

== system halout/HAL_OUT/CAN1/FD_APS1_0x236 ==
  BSCP_outputs : Inport  OutDataTypeStr=Bus: BSCP_outputs
  BOUTP_outputs : Inport  Port=2  OutDataTypeStr=Bus: BOUTP_outputs
  APSAngleTarget : Subsystem
  APSRqEPASCtrl : Subsystem
  APSStaSystem : Subsystem
  APSVRqEPASCtrl : Subsystem
  bus_creator : BusCreator  Inputs=4  OutDataTypeStr=Bus: DT_CAN1_SG_FD_APS1  NonVirtualBus=on
  bus_selector : BusSelector  OutputSignals=VOUTP_APSAngleTarget_Deg
  bus_selector1 : BusSelector  OutputSignals=VOUTP_APSRqEPASCtrl_flg
  bus_selector2 : BusSelector  OutputSignals=VOUTP_APSStaSys_enum
  bus_selector3 : BusSelector  OutputSignals=VOUTP_APSVRqEPASCtrl_flg
  FD_APS1 : Outport
  wires:
  BSCP_outputs/1 -> [BSCP_outputs]
  BOUTP_outputs/1 -> [BOUTP_outputs]
  [CAN1_APS_Angle_Target] -> bus_creator/1  "CAN1_APS_Angle_Target"
  [CAN1_APS_Rq_EPAS_Ctrl] -> bus_creator/2  "CAN1_APS_Rq_EPAS_Ctrl"
  [CAN1_APS_Sta_System] -> bus_creator/3  "CAN1_APS_Sta_System"
  [CAN1_APS_V_Rq_EPAS_Ctrl] -> bus_creator/4  "CAN1_APS_V_Rq_EPAS_Ctrl"
  bus_creator/1 -> FD_APS1/1
  APSAngleTarget/1(CAN1_APS_Angle_Target) -> [CAN1_APS_Angle_Target]
  APSRqEPASCtrl/1(CAN1_APS_Rq_EPAS_Ctrl) -> [CAN1_APS_Rq_EPAS_Ctrl]
  APSStaSystem/1(CAN1_APS_Sta_System) -> [CAN1_APS_Sta_System]
  APSVRqEPASCtrl/1(CAN1_APS_V_Rq_EPAS_Ctrl) -> [CAN1_APS_V_Rq_EPAS_Ctrl]
  bus_selector/1 -> APSAngleTarget/1(APSAngleTarget)  "<VOUTP_APSAngleTarget_Deg>"
  [BOUTP_outputs] -> bus_selector/1
  bus_selector1/1 -> APSRqEPASCtrl/1(APSRqEPASCtrl)  "<VOUTP_APSRqEPASCtrl_flg>"
  [BOUTP_outputs] -> bus_selector1/1
  bus_selector2/1 -> APSStaSystem/1(APSStaSystem)  "<VOUTP_APSStaSys_enum>"
  [BOUTP_outputs] -> bus_selector2/1
  bus_selector3/1 -> APSVRqEPASCtrl/1(APSVRqEPASCtrl)  "<VOUTP_APSVRqEPASCtrl_flg>"
  [BOUTP_outputs] -> bus_selector3/1

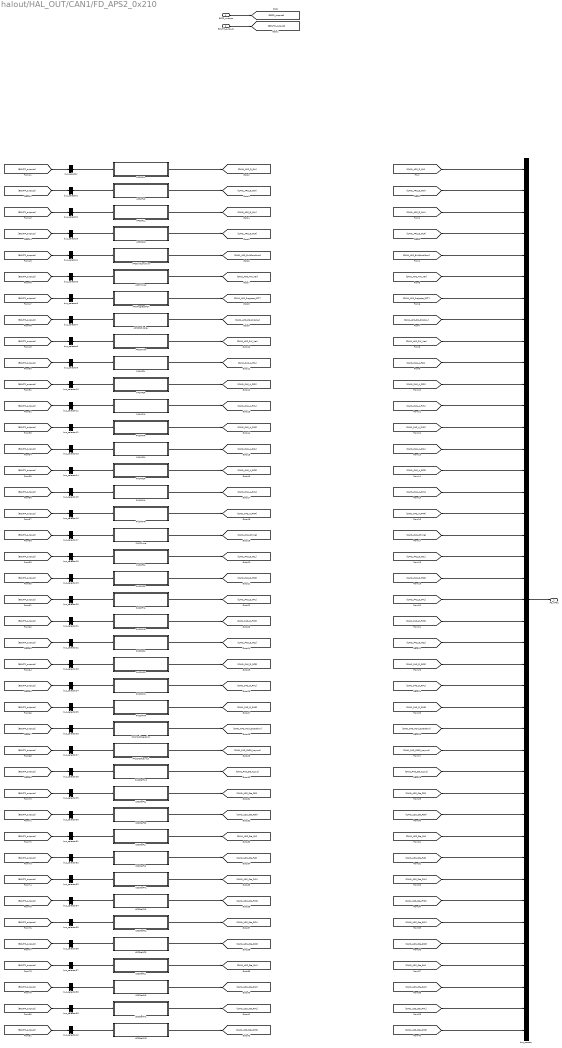
== system halout/HAL_OUT/CAN1/FD_APS2_0x210 ==
  BSCP_outputs : Inport  OutDataTypeStr=Bus: BSCP_outputs
  BOUTP_outputs : Inport  Port=2  OutDataTypeStr=Bus: BOUTP_outputs
  APSDFLL : Subsystem
  APSDFLR : Subsystem
  APSDRLL : Subsystem
  APSDRLR : Subsystem
  APSExitCondition : Subsystem
  APSHWVer : Subsystem
  APSProgressPCT : Subsystem
  APSRQDisplay : Subsystem
  APSSWVer : Subsystem
  PASAFCL : Subsystem
  PASAFCR : Subsystem
  PASAFML : Subsystem
  PASAFMR : Subsystem
  PASARCL : Subsystem
  PASARCR : Subsystem
  PASARML : Subsystem
  PASARMR : Subsystem
  PASChime : Subsystem
  PASDFCL : Subsystem
  PASDFCR : Subsystem
  PASDFML : Subsystem
  PASDFMR : Subsystem
  PASDRCL : Subsystem
  PASDRCR : Subsystem
  PASDRML : Subsystem
  PASDRMR : Subsystem
  PASModOperation : Subsystem
  PASSNSRLayout : Subsystem
  PASStaFSys : Subsystem
  USSStaFCL : Subsystem
  USSStaFCR : Subsystem
  USSStaFLL : Subsystem
  USSStaFLR : Subsystem
  USSStaFML : Subsystem
  USSStaFMR : Subsystem
  USSStaRCL : Subsystem
  USSStaRCR : Subsystem
  USSStaRLL : Subsystem
  USSStaRLR : Subsystem
  USSStaRML : Subsystem
  USSStaRMR : Subsystem
  bus_creator : BusCreator  Inputs=41  OutDataTypeStr=Bus: DT_CAN1_SG_FD_APS2  NonVirtualBus=on
  bus_selector : BusSelector  OutputSignals=VOUTP_APSDFLL_cm
  bus_selector1 : BusSelector  OutputSignals=VOUTP_APSDFLR_cm
  bus_selector10 : BusSelector  OutputSignals=VOUTP_PASAFCR_enum
  bus_selector11 : BusSelector  OutputSignals=VOUTP_PASAFML_enum
  bus_selector12 : BusSelector  OutputSignals=VOUTP_PASAFMR_enum
  bus_selector13 : BusSelector  OutputSignals=VOUTP_PASARCL_enum
  bus_selector14 : BusSelector  OutputSignals=VOUTP_PASARCR_enum
  bus_selector15 : BusSelector  OutputSignals=VOUTP_PASARML_enum
  bus_selector16 : BusSelector  OutputSignals=VOUTP_PASARMR_enum
  bus_selector17 : BusSelector  OutputSignals=VOUTP_Chime_enum
  bus_selector18 : BusSelector  OutputSignals=VOUTP_PASDFCL_cm
  bus_selector19 : BusSelector  OutputSignals=VOUTP_PASDFCR_cm
  bus_selector2 : BusSelector  OutputSignals=VOUTP_APSDRLL_cm
  bus_selector20 : BusSelector  OutputSignals=VOUTP_PASDFML_cm
  bus_selector21 : BusSelector  OutputSignals=VOUTP_PASDFMR_cm
  bus_selector22 : BusSelector  OutputSignals=VOUTP_PASDRCL_cm
  bus_selector23 : BusSelector  OutputSignals=VOUTP_PASDRCR_cm
  bus_selector24 : BusSelector  OutputSignals=VOUTP_PASDRML_cm
  bus_selector25 : BusSelector  OutputSignals=VOUTP_PASDRMR_cm
  bus_selector26 : BusSelector  OutputSignals=VOUTP_ModOperation_enum
  bus_selector27 : BusSelector  OutputSignals=VOUTP_SNSRLayout_enum
  bus_selector28 : BusSelector  OutputSignals=VOUTP_StaFSya_flg
  bus_selector29 : BusSelector  OutputSignals=VOUTP_USSStaFCL_flg
  bus_selector3 : BusSelector  OutputSignals=VOUTP_APSDRLR_cm
  bus_selector30 : BusSelector  OutputSignals=VOUTP_USSStaFCR_flg
  bus_selector31 : BusSelector  OutputSignals=VOUTP_USSStaFLL_flg
  bus_selector32 : BusSelector  OutputSignals=VOUTP_USSStaFLR_flg
  bus_selector33 : BusSelector  OutputSignals=VOUTP_USSStaFML_flg
  bus_selector34 : BusSelector  OutputSignals=VOUTP_USSStaFMR_flg
  bus_selector35 : BusSelector  OutputSignals=VOUTP_USSStaRCL_flg
  bus_selector36 : BusSelector  OutputSignals=VOUTP_USSStaRCR_flg
  bus_selector37 : BusSelector  OutputSignals=VOUTP_USSStaRLL_flg
  bus_selector38 : BusSelector  OutputSignals=VOUTP_USSStaRLR_flg
  bus_selector39 : BusSelector  OutputSignals=VOUTP_USSStaRML_flg
  bus_selector4 : BusSelector  OutputSignals=VOUTP_APSExitCondition_enum
  bus_selector40 : BusSelector  OutputSignals=VOUTP_USSStaRMR_flg
  bus_selector5 : BusSelector  OutputSignals=VOUTP_APSHWVer_enum
  bus_selector6 : BusSelector  OutputSignals=VOUTP_APSProgressPCT_pct
  bus_selector7 : BusSelector  OutputSignals=VOUTP_APSRQDisplay_enum
  bus_selector8 : BusSelector  OutputSignals=VOUTP_APSSWVer_enum
  bus_selector9 : BusSelector  OutputSignals=VOUTP_PASAFCL_enum
  FD_APS2 : Outport
  wires:
  BSCP_outputs/1 -> [BSCP_outputs]
  BOUTP_outputs/1 -> [BOUTP_outputs]
  [CAN1_APS_D_FLL] -> bus_creator/1  "CAN1_APS_D_FLL"
  [CAN1_APS_D_FLR] -> bus_creator/2  "CAN1_APS_D_FLR"
  [CAN1_APS_D_RLL] -> bus_creator/3  "CAN1_APS_D_RLL"
  [CAN1_APS_D_RLR] -> bus_creator/4  "CAN1_APS_D_RLR"
  [CAN1_APS_ExitCondition] -> bus_creator/5  "CAN1_APS_ExitCondition"
  [CAN1_APS_HW_Ver] -> bus_creator/6  "CAN1_APS_HW_Ver"
  [CAN1_APS_Progress_PCT] -> bus_creator/7  "CAN1_APS_Progress_PCT"
  [CAN1_APS_RQ_Display] -> bus_creator/8  "CAN1_APS_RQ_Display"
  [CAN1_APS_SW_Ver] -> bus_creator/9  "CAN1_APS_SW_Ver"
  [CAN1_PAS_A_FCL] -> bus_creator/10  "CAN1_PAS_A_FCL"
  [CAN1_PAS_A_FCR] -> bus_creator/11  "CAN1_PAS_A_FCR"
  [CAN1_PAS_A_FML] -> bus_creator/12  "CAN1_PAS_A_FML"
  [CAN1_PAS_A_FMR] -> bus_creator/13  "CAN1_PAS_A_FMR"
  [CAN1_PAS_A_RCL] -> bus_creator/14  "CAN1_PAS_A_RCL"
  [CAN1_PAS_A_RCR] -> bus_creator/15  "CAN1_PAS_A_RCR"
  [CAN1_PAS_A_RML] -> bus_creator/16  "CAN1_PAS_A_RML"
  [CAN1_PAS_A_RMR] -> bus_creator/17  "CAN1_PAS_A_RMR"
  [CAN1_PAS_Chime] -> bus_creator/18  "CAN1_PAS_Chime"
  [CAN1_PAS_D_FCL] -> bus_creator/19  "CAN1_PAS_D_FCL"
  [CAN1_PAS_D_FCR] -> bus_creator/20  "CAN1_PAS_D_FCR"
  [CAN1_PAS_D_FML] -> bus_creator/21  "CAN1_PAS_D_FML"
  [CAN1_PAS_D_FMR] -> bus_creator/22  "CAN1_PAS_D_FMR"
  [CAN1_PAS_D_RCL] -> bus_creator/23  "CAN1_PAS_D_RCL"
  [CAN1_PAS_D_RCR] -> bus_creator/24  "CAN1_PAS_D_RCR"
  [CAN1_PAS_D_RML] -> bus_creator/25  "CAN1_PAS_D_RML"
  [CAN1_PAS_D_RMR] -> bus_creator/26  "CAN1_PAS_D_RMR"
  [CAN1_PAS_Mod_Operation] -> bus_creator/27  "CAN1_PAS_Mod_Operation"
  [CAN1_PAS_SNSR_Layout] -> bus_creator/28  "CAN1_PAS_SNSR_Layout"
  [CAN1_PAS_Sta_F_Sys] -> bus_creator/29  "CAN1_PAS_Sta_F_Sys"
  [CAN1_USS_Sta_FCL] -> bus_creator/30  "CAN1_USS_Sta_FCL"
  [CAN1_USS_Sta_FCR] -> bus_creator/31  "CAN1_USS_Sta_FCR"
  [CAN1_USS_Sta_FLL] -> bus_creator/32  "CAN1_USS_Sta_FLL"
  [CAN1_USS_Sta_FLR] -> bus_creator/33  "CAN1_USS_Sta_FLR"
  [CAN1_USS_Sta_FML] -> bus_creator/34  "CAN1_USS_Sta_FML"
  [CAN1_USS_Sta_FMR] -> bus_creator/35  "CAN1_USS_Sta_FMR"
  [CAN1_USS_Sta_RCL] -> bus_creator/36  "CAN1_USS_Sta_RCL"
  [CAN1_USS_Sta_RCR] -> bus_creator/37  "CAN1_USS_Sta_RCR"
  [CAN1_USS_Sta_RLL] -> bus_creator/38  "CAN1_USS_Sta_RLL"
  [CAN1_USS_Sta_RLR] -> bus_creator/39  "CAN1_USS_Sta_RLR"
  [CAN1_USS_Sta_RML] -> bus_creator/40  "CAN1_USS_Sta_RML"
  [CAN1_USS_Sta_RMR] -> bus_creator/41  "CAN1_USS_Sta_RMR"
  bus_creator/1 -> FD_APS2/1
  APSDFLL/1(CAN1_APS_D_FLL) -> [CAN1_APS_D_FLL]
  APSDFLR/1(CAN1_APS_D_FLR) -> [CAN1_APS_D_FLR]
  APSDRLL/1(CAN1_APS_D_RLL) -> [CAN1_APS_D_RLL]
  APSDRLR/1(CAN1_APS_D_RLR) -> [CAN1_APS_D_RLR]
  APSExitCondition/1(CAN1_APS_ExitCondition) -> [CAN1_APS_ExitCondition]
  APSHWVer/1(CAN1_APS_HW_Ver) -> [CAN1_APS_HW_Ver]
  APSProgressPCT/1(CAN1_APS_Progress_PCT) -> [CAN1_APS_Progress_PCT]
  APSRQDisplay/1(CAN1_APS_RQ_Display) -> [CAN1_APS_RQ_Display]
  APSSWVer/1(CAN1_APS_SW_Ver) -> [CAN1_APS_SW_Ver]
  PASAFCL/1(CAN1_PAS_A_FCL) -> [CAN1_PAS_A_FCL]
  PASAFCR/1(CAN1_PAS_A_FCR) -> [CAN1_PAS_A_FCR]
  PASAFML/1(CAN1_PAS_A_FML) -> [CAN1_PAS_A_FML]
  PASAFMR/1(CAN1_PAS_A_FMR) -> [CAN1_PAS_A_FMR]
  PASARCL/1(CAN1_PAS_A_RCL) -> [CAN1_PAS_A_RCL]
  PASARCR/1(CAN1_PAS_A_RCR) -> [CAN1_PAS_A_RCR]
  PASARML/1(CAN1_PAS_A_RML) -> [CAN1_PAS_A_RML]
  PASARMR/1(CAN1_PAS_A_RMR) -> [CAN1_PAS_A_RMR]
  PASChime/1(CAN1_PAS_Chime) -> [CAN1_PAS_Chime]
  PASDFCL/1(CAN1_PAS_D_FCL) -> [CAN1_PAS_D_FCL]
  PASDFCR/1(CAN1_PAS_D_FCR) -> [CAN1_PAS_D_FCR]
  PASDFML/1(CAN1_PAS_D_FML) -> [CAN1_PAS_D_FML]
  PASDFMR/1(CAN1_PAS_D_FMR) -> [CAN1_PAS_D_FMR]
  PASDRCL/1(CAN1_PAS_D_RCL) -> [CAN1_PAS_D_RCL]
  PASDRCR/1(CAN1_PAS_D_RCR) -> [CAN1_PAS_D_RCR]
  PASDRML/1(CAN1_PAS_D_RML) -> [CAN1_PAS_D_RML]
  PASDRMR/1(CAN1_PAS_D_RMR) -> [CAN1_PAS_D_RMR]
  PASModOperation/1(CAN1_PAS_Mod_Operation) -> [CAN1_PAS_Mod_Operation]
  PASSNSRLayout/1(CAN1_PAS_SNSR_Layout) -> [CAN1_PAS_SNSR_Layout]
  PASStaFSys/1(CAN1_PAS_Sta_F_Sys) -> [CAN1_PAS_Sta_F_Sys]
  USSStaFCL/1(CAN1_USS_Sta_FCL) -> [CAN1_USS_Sta_FCL]
  USSStaFCR/1(CAN1_USS_Sta_FCR) -> [CAN1_USS_Sta_FCR]
  USSStaFLL/1(CAN1_USS_Sta_FLL) -> [CAN1_USS_Sta_FLL]
  USSStaFLR/1(CAN1_USS_Sta_FLR) -> [CAN1_USS_Sta_FLR]
  USSStaFML/1(CAN1_USS_Sta_FML) -> [CAN1_USS_Sta_FML]
  USSStaFMR/1(CAN1_USS_Sta_FMR) -> [CAN1_USS_Sta_FMR]
  USSStaRCL/1(CAN1_USS_Sta_RCL) -> [CAN1_USS_Sta_RCL]
  USSStaRCR/1(CAN1_USS_Sta_RCR) -> [CAN1_USS_Sta_RCR]
  USSStaRLL/1(CAN1_USS_Sta_RLL) -> [CAN1_USS_Sta_RLL]
  USSStaRLR/1(CAN1_USS_Sta_RLR) -> [CAN1_USS_Sta_RLR]
  USSStaRML/1(CAN1_USS_Sta_RML) -> [CAN1_USS_Sta_RML]
  USSStaRMR/1(CAN1_USS_Sta_RMR) -> [CAN1_USS_Sta_RMR]
  bus_selector/1 -> APSDFLL/1(APSDFLL)  "<VOUTP_APSDFLL_cm>"
  [BOUTP_outputs] -> bus_selector/1
  bus_selector1/1 -> APSDFLR/1(APSDFLR)  "<VOUTP_APSDFLR_cm>"
  [BOUTP_outputs] -> bus_selector1/1
  bus_selector2/1 -> APSDRLL/1(APSDRLL)  "<VOUTP_APSDRLL_cm>"
  [BOUTP_outputs] -> bus_selector2/1
  bus_selector3/1 -> APSDRLR/1(APSDRLR)  "<VOUTP_APSDRLR_cm>"
  [BOUTP_outputs] -> bus_selector3/1
  bus_selector4/1 -> APSExitCondition/1(APSExitCondition)  "<VOUTP_APSExitCondition_enum>"
  [BOUTP_outputs] -> bus_selector4/1
  bus_selector5/1 -> APSHWVer/1(APSHWVer)  "<VOUTP_APSHWVer_enum>"
  [BOUTP_outputs] -> bus_selector5/1
  bus_selector6/1 -> APSProgressPCT/1(APSProgressPCT)  "<VOUTP_APSProgressPCT_pct>"
  [BOUTP_outputs] -> bus_selector6/1
  bus_selector7/1 -> APSRQDisplay/1(APSRQDisplay)  "<VOUTP_APSRQDisplay_enum>"
  [BOUTP_outputs] -> bus_selector7/1
  bus_selector8/1 -> APSSWVer/1(APSSWVer)  "<VOUTP_APSSWVer_enum>"
  [BOUTP_outputs] -> bus_selector8/1
  bus_selector9/1 -> PASAFCL/1(PASAFCL)  "<VOUTP_PASAFCL_enum>"
  [BOUTP_outputs] -> bus_selector9/1
  bus_selector10/1 -> PASAFCR/1(PASAFCR)  "<VOUTP_PASAFCR_enum>"
  [BOUTP_outputs] -> bus_selector10/1
  bus_selector11/1 -> PASAFML/1(PASAFML)  "<VOUTP_PASAFML_enum>"
  [BOUTP_outputs] -> bus_selector11/1
  bus_selector12/1 -> PASAFMR/1(PASAFMR)  "<VOUTP_PASAFMR_enum>"
  [BOUTP_outputs] -> bus_selector12/1
  bus_selector13/1 -> PASARCL/1(PASARCL)  "<VOUTP_PASARCL_enum>"
  [BOUTP_outputs] -> bus_selector13/1
  bus_selector14/1 -> PASARCR/1(PASARCR)  "<VOUTP_PASARCR_enum>"
  [BOUTP_outputs] -> bus_selector14/1
  bus_selector15/1 -> PASARML/1(PASARML)  "<VOUTP_PASARML_enum>"
  [BOUTP_outputs] -> bus_selector15/1
  bus_selector16/1 -> PASARMR/1(PASARMR)  "<VOUTP_PASARMR_enum>"
  [BOUTP_outputs] -> bus_selector16/1
  bus_selector17/1 -> PASChime/1(PASChime)  "<VOUTP_Chime_enum>"
  [BOUTP_outputs] -> bus_selector17/1
  bus_selector18/1 -> PASDFCL/1(PASDFCL)  "<VOUTP_PASDFCL_cm>"
  [BOUTP_outputs] -> bus_selector18/1
  bus_selector19/1 -> PASDFCR/1(PASDFCR)  "<VOUTP_PASDFCR_cm>"
  [BOUTP_outputs] -> bus_selector19/1
  bus_selector20/1 -> PASDFML/1(PASDFML)  "<VOUTP_PASDFML_cm>"
  [BOUTP_outputs] -> bus_selector20/1
  bus_selector21/1 -> PASDFMR/1(PASDFMR)  "<VOUTP_PASDFMR_cm>"
  [BOUTP_outputs] -> bus_selector21/1
  bus_selector22/1 -> PASDRCL/1(PASDRCL)  "<VOUTP_PASDRCL_cm>"
  [BOUTP_outputs] -> bus_selector22/1
  bus_selector23/1 -> PASDRCR/1(PASDRCR)  "<VOUTP_PASDRCR_cm>"
  [BOUTP_outputs] -> bus_selector23/1
  bus_selector24/1 -> PASDRML/1(PASDRML)  "<VOUTP_PASDRML_cm>"
  [BOUTP_outputs] -> bus_selector24/1
  bus_selector25/1 -> PASDRMR/1(PASDRMR)  "<VOUTP_PASDRMR_cm>"
  [BOUTP_outputs] -> bus_selector25/1
  bus_selector26/1 -> PASModOperation/1(PASModOperation)  "<VOUTP_ModOperation_enum>"
  [BOUTP_outputs] -> bus_selector26/1
  bus_selector27/1 -> PASSNSRLayout/1(PASSNSRLayout)  "<VOUTP_SNSRLayout_enum>"
  [BOUTP_outputs] -> bus_selector27/1
  bus_selector28/1 -> PASStaFSys/1(PASStaFSys)  "<VOUTP_StaFSya_flg>"
  [BOUTP_outputs] -> bus_selector28/1
  bus_selector29/1 -> USSStaFCL/1(USSStaFCL)  "<VOUTP_USSStaFCL_flg>"
  [BOUTP_outputs] -> bus_selector29/1
  bus_selector30/1 -> USSStaFCR/1(USSStaFCR)  "<VOUTP_USSStaFCR_flg>"
  [BOUTP_outputs] -> bus_selector30/1
  bus_selector31/1 -> USSStaFLL/1(USSStaFLL)  "<VOUTP_USSStaFLL_flg>"
  [BOUTP_outputs] -> bus_selector31/1
  bus_selector32/1 -> USSStaFLR/1(USSStaFLR)  "<VOUTP_USSStaFLR_flg>"
  [BOUTP_outputs] -> bus_selector32/1
  bus_selector33/1 -> USSStaFML/1(USSStaFML)  "<VOUTP_USSStaFML_flg>"
  [BOUTP_outputs] -> bus_selector33/1
  bus_selector34/1 -> USSStaFMR/1(USSStaFMR)  "<VOUTP_USSStaFMR_flg>"
  [BOUTP_outputs] -> bus_selector34/1
  bus_selector35/1 -> USSStaRCL/1(USSStaRCL)  "<VOUTP_USSStaRCL_flg>"
  [BOUTP_outputs] -> bus_selector35/1
  bus_selector36/1 -> USSStaRCR/1(USSStaRCR)  "<VOUTP_USSStaRCR_flg>"
  [BOUTP_outputs] -> bus_selector36/1
  bus_selector37/1 -> USSStaRLL/1(USSStaRLL)  "<VOUTP_USSStaRLL_flg>"
  [BOUTP_outputs] -> bus_selector37/1
  bus_selector38/1 -> USSStaRLR/1(USSStaRLR)  "<VOUTP_USSStaRLR_flg>"
  [BOUTP_outputs] -> bus_selector38/1
  bus_selector39/1 -> USSStaRML/1(USSStaRML)  "<VOUTP_USSStaRML_flg>"
  [BOUTP_outputs] -> bus_selector39/1
  bus_selector40/1 -> USSStaRMR/1(USSStaRMR)  "<VOUTP_USSStaRMR_flg>"
  [BOUTP_outputs] -> bus_selector40/1

== system halout/HAL_OUT/CAN1/FD_APS3_0x238 ==
  BSCP_outputs : Inport  OutDataTypeStr=Bus: BSCP_outputs
  BOUTP_outputs : Inport  Port=2  OutDataTypeStr=Bus: BOUTP_outputs
  Trigger : TriggerPort  TriggerType=function-call  VariantControl=(inherit)
  APS3LifeCount : Subsystem
  APS3checksum : Subsystem
  APSDecReq : Subsystem
  APSDecReqA : Subsystem
  APSOpenPTG : Subsystem
  APSReq : Subsystem
  Byte_0 : Subsystem
  Byte_1 : Subsystem
  Byte_2 : Subsystem
  Byte_3 : Constant  Value=ZERO_INT
  Byte_4 : Constant  Value=ZERO_INT
  Byte_5 : Constant  Value=ZERO_INT
  Byte_6 : Subsystem
  Byte_7 : Subsystem
  CAASSta : Subsystem
  CRC8_IfAction_Tx : FVT_lib/hal/CRC8_IfAction_Tx
  Constant : Constant  Value=KHAL_CAN1FDAPS3E2E_flg
  Constant1 : Constant  Value=0x00
  Constant2 : Constant  Value=0x00
  Constant3 : Constant  Value=KHAL_CAN1FDAPS3E2E_flg
  Constant4 : Constant  Value=KHAL_CAN1FDAPS3E2E_flg
  Ground : Ground
  Ground1 : Ground
  Ground2 : Ground
  Mux2 : Mux  Inputs=7
  RollingCounter_IfAction : FVT_lib/hal/RollingCounter_IfAction
  RollingCounter_IfAction1 : FVT_lib/hal/RollingCounter_IfAction
  SPTGDet : Subsystem
  SPTGSta : Subsystem
  Terminator : Terminator
  bus_creator : BusCreator  Inputs=9  OutDataTypeStr=Bus: DT_CAN1_SG_FD_APS3  NonVirtualBus=on
  bus_selector : BusSelector  OutputSignals=VOUTP_APSOpenPTG_flg
  bus_selector1 : BusSelector  OutputSignals=VOUTP_APSDecReqA_flg
  bus_selector10 : BusSelector  OutputSignals=VOUTP_CAASSta_enum
  bus_selector11 : BusSelector  OutputSignals=VOUTP_SPTGDet_flg
  bus_selector2 : BusSelector  OutputSignals=VOUTP_CAASSta_enum
  bus_selector3 : BusSelector  OutputSignals=VOUTP_SPTGDet_flg
  bus_selector4 : BusSelector  OutputSignals=VOUTP_APSDecReq_mps2
  bus_selector5 : BusSelector  OutputSignals=VOUTP_APSReq_enum
  bus_selector6 : BusSelector  OutputSignals=VOUTP_APSOpenPTG_flg
  bus_selector7 : BusSelector  OutputSignals=VOUTP_APSDecReq_mps2
  bus_selector8 : BusSelector  OutputSignals=VOUTP_APSDecReqA_flg
  bus_selector9 : BusSelector  OutputSignals=VOUTP_APSReq_enum
  FD_APS3 : Outport
  wires:
  BSCP_outputs/1 -> [BSCP_outputs]
  BOUTP_outputs/1 -> [BOUTP_outputs]
  [CAN1_APS3_LifeCount] -> bus_creator/1  "CAN1_APS3_LifeCount"
  [CAN1_APS3_checksum] -> bus_creator/2  "CAN1_APS3_checksum"
  [CAN1_APSOpenPTG] -> bus_creator/3  "CAN1_APSOpenPTG"
  [CAN1_APS_DecReq] -> bus_creator/4  "CAN1_APS_DecReq"
  [CAN1_APS_DecReq_A] -> bus_creator/5  "CAN1_APS_DecReq_A"
  [CAN1_APS_Req] -> bus_creator/6  "CAN1_APS_Req"
  [CAN1_CAAS_Sta] -> bus_creator/7  "CAN1_CAAS_Sta"
  [CAN1_SPTGDet] -> bus_creator/8  "CAN1_SPTGDet"
  [CAN1_SPTG_Sta] -> bus_creator/9  "CAN1_SPTG_Sta"
  bus_creator/1 -> FD_APS3/1
  APS3LifeCount/1(CAN1_APS3_LifeCount) -> [CAN1_APS3_LifeCount]
  APS3checksum/1(CAN1_APS3_checksum) -> [CAN1_APS3_checksum]
  APSOpenPTG/1(CAN1_APSOpenPTG) -> [CAN1_APSOpenPTG]
  APSDecReq/1(CAN1_APS_DecReq) -> [CAN1_APS_DecReq]
  APSDecReqA/1(CAN1_APS_DecReq_A) -> [CAN1_APS_DecReq_A]
  APSReq/1(CAN1_APS_Req) -> [CAN1_APS_Req]
  CAASSta/1(CAN1_CAAS_Sta) -> [CAN1_CAAS_Sta]
  SPTGDet/1(CAN1_SPTGDet) -> [CAN1_SPTGDet]
  SPTGSta/1(CAN1_SPTG_Sta) -> [CAN1_SPTG_Sta]
  Byte_0/1(Byte_0) -> [Byte_0]
  Byte_1/1(Byte_1) -> [Byte_1]
  Byte_2/1(Byte_2) -> [Byte_2]
  Byte_3/1 -> [Byte_3]
  Byte_4/1 -> [Byte_4]
  Byte_5/1 -> [Byte_5]
  Byte_6/1(Byte_6) -> [Byte_6]
  Byte_7/1(Byte_7) -> Terminator/1
  Mux2/1 -> CRC8_IfAction_Tx/4
  Constant/1 -> CRC8_IfAction_Tx/1
  Constant1/1 -> CRC8_IfAction_Tx/2
  Constant2/1 -> CRC8_IfAction_Tx/3
  CRC8_IfAction_Tx/1 -> [APS3_checksum]
  [Byte_0] -> Mux2/1
  bus_selector/1 -> Byte_0/1(APSOpenPTG)  "<VOUTP_APSOpenPTG_flg>"
  [BOUTP_outputs] -> bus_selector/1
  bus_selector1/1 -> Byte_0/2(APS_DecReq_A)  "<VOUTP_APSDecReqA_flg>"
  [BOUTP_outputs] -> bus_selector1/1
  bus_selector2/1 -> Byte_0/3(CAAS_Sta)  "<VOUTP_CAASSta_enum>"
  [BOUTP_outputs] -> bus_selector2/1
  bus_selector3/1 -> Byte_0/4(SPTGDet)  "<VOUTP_SPTGDet_flg>"
  [BOUTP_outputs] -> bus_selector3/1
  [Byte_1] -> Mux2/2
  bus_selector4/1 -> Byte_1/1(APS_DecReq)  "<VOUTP_APSDecReq_mps2>"
  [BOUTP_outputs] -> bus_selector4/1
  [Byte_2] -> Mux2/3
  bus_selector5/1 -> Byte_2/1(APS_Req)  "<VOUTP_APSReq_enum>"
  [BOUTP_outputs] -> bus_selector5/1
  Ground/1 -> Byte_2/2(SPTG_Sta)
  [Byte_3] -> Mux2/4
  [Byte_4] -> Mux2/5
  [Byte_5] -> Mux2/6
  [Byte_6] -> Mux2/7
  RollingCounter_IfAction/1 -> Byte_6/1(APS3_LifeCount)
  Constant3/1 -> RollingCounter_IfAction/1
  Ground1/1 -> Byte_7/1(APS3_checksum)
  RollingCounter_IfAction1/1 -> APS3LifeCount/1(APS3LifeCount)
  Constant4/1 -> RollingCounter_IfAction1/1
  [APS3_checksum] -> APS3checksum/1(APS3checksum)
  bus_selector6/1 -> APSOpenPTG/1(APSOpenPTG)  "<VOUTP_APSOpenPTG_flg>"
  [BOUTP_outputs] -> bus_selector6/1
  bus_selector7/1 -> APSDecReq/1(APSDecReq)  "<VOUTP_APSDecReq_mps2>"
  [BOUTP_outputs] -> bus_selector7/1
  bus_selector8/1 -> APSDecReqA/1(APSDecReqA)  "<VOUTP_APSDecReqA_flg>"
  [BOUTP_outputs] -> bus_selector8/1
  bus_selector9/1 -> APSReq/1(APSReq)  "<VOUTP_APSReq_enum>"
  [BOUTP_outputs] -> bus_selector9/1
  bus_selector10/1 -> CAASSta/1(CAASSta)  "<VOUTP_CAASSta_enum>"
  [BOUTP_outputs] -> bus_selector10/1
  bus_selector11/1 -> SPTGDet/1(SPTGDet)  "<VOUTP_SPTGDet_flg>"
  [BOUTP_outputs] -> bus_selector11/1
  Ground2/1 -> SPTGSta/1(SPTGSta)

== system halout/HAL_OUT/CAN1/FD_APS3_Tx ==
  TxReq : Inport
  Chart : Stateflow chart  TreatAsAtomicUnit=on
  Constant : Constant  Value=C_TASK_5MS_S
  Constant3 : Constant  Value=CycleTime
  Data Type Conversion : DataTypeConversion  OutDataTypeStr=uint16
  Divide : Product  Inputs=*/
  Gain : Gain  Gain=0.001
  TxTrigger : Outport
  wires:
  Data Type Conversion/1 -> Chart/2(CycleCnt)
  Constant3/1 -> Gain/1
  Gain/1 -> Divide/1
  Chart/1(TxTrigger()) -> TxTrigger/1
  Divide/1 -> Data Type Conversion/1
  TxReq/1 -> Chart/1(TxReq)
  Constant/1 -> Divide/2
